simulink model "LQR_Hardware"  (R2022b)
settings: Solver=ode1  StartTime=0.0  StopTime=inf  FixedStep=0.001  RelTol=1e-3
values from neighbouring files (symbols this model uses):
  KK = lqr(A,B,Q,R)    [Init_Setup_LQRArd.m]    (also in Parameters.m)
libraries: arduinolib x4, arduinosensorlib x2
settings Model: ExtModeTrigDuration=2  Creator=sokse  LastModifiedBy=sokse
settings OptimizationCC: EnhancedBackFolding=on  PassReuseOutputArgsAs=Individual arguments  ZeroExternalMemoryAtStartup=off  ZeroInternalMemoryAtStartup=off  MaxStackSize=64  OptimizeBlockOrder=speed  DifferentSizesBufferReuse=on  OptimizationCustomize=off  EfficientTunableParamExpr=on
settings DebuggingCC: ParameterTunabilityLossMsg=error
settings HardwareCC: ProdBitPerInt=16  ProdBitPerPointer=16  ProdBitPerSizeT=16  ProdBitPerPtrDiffT=16  ProdLargestAtomicFloat=None  ProdWordSize=8  ProdHWDeviceType=Atmel->AVR
settings SFSimCC: MATLABDynamicMemAlloc=off
settings RTWCC: Description=Embedded Coder  SystemTargetFile=ert.tlc  HardwareBoard=Arduino Mega 2560  TLCOptions=-aInlineSetEventsForThisBaseRateFcn=TLC_FALSE -aSuppressMultiTaskScheduler=TLC_FALSE -aRateBasedStepFcn=1  TemplateMakefile=ert_default_tmf  Toolchain=Arduino AVR  BuildConfiguration=Faster Runs
settings CodeAppCC: ForceParamTrailComments=on  IgnoreCustomStorageClasses=off  OperatorAnnotations=on  SimulinkDataObjDesc=on  SFDataObjDesc=on  InsertBlockDesc=on
settings ERTTargetCC: SupportContinuousTime=on  SupportVariableSizeSignals=on  ExtModeTransport=3  ExtModeStaticAlloc=on  ExtModeAutomaticAllocSize=off  ExtModeStaticAllocSize=2048  ExtModeMexFile=ext_xcp  ExtModeIntrfLevel=Level2 - Open

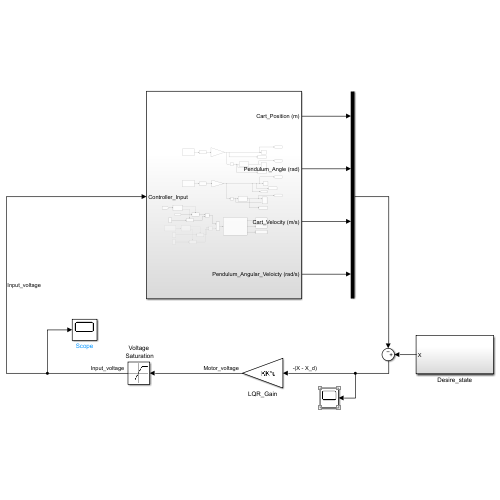
[thumbnail: Simulink's stored preview of the top-level diagram]
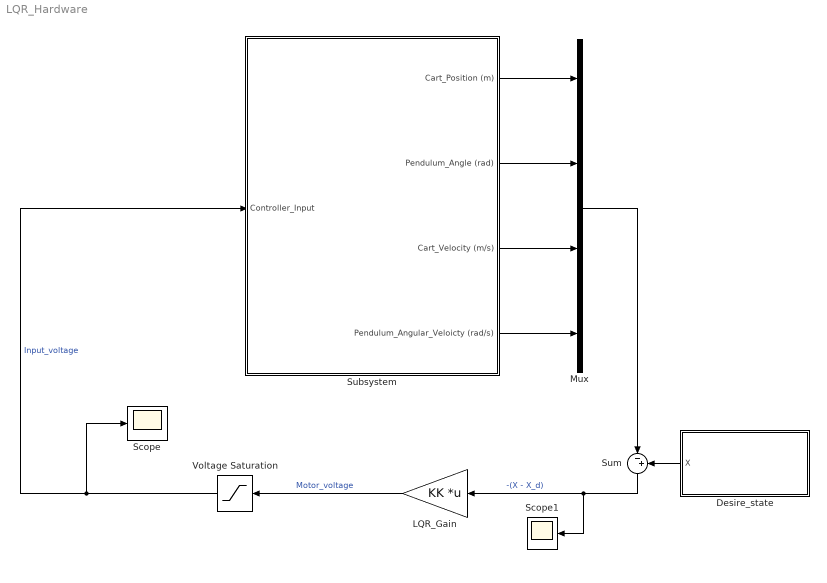
== system LQR_Hardware ==
  Desire_state : Subsystem
  LQR_Gain : Gain  Gain=KK  Multiplication=Matrix(K*u)
  Mux : Mux
  Scope : Scope
  Scope1 : Scope
  Subsystem : Subsystem
  Sum : Sum  Inputs=|-+
  Voltage Saturation : Saturate  UpperLimit=12  LowerLimit=-12
  wires:
  Voltage Saturation/1 -> Scope/1, Subsystem/1(Controller_Input)  "Input_voltage"
  Sum/1 -> Scope1/1, LQR_Gain/1  "-(X - X_d)"
  Desire_state/1(X) -> Sum/2
  LQR_Gain/1 -> Voltage Saturation/1  "Motor_voltage"
  Subsystem/1(Cart_Position (m)) -> Mux/1
  Subsystem/2(Pendulum_Angle (rad)) -> Mux/2
  Subsystem/3(Cart_Velocity (m/s)) -> Mux/3
  Subsystem/4(Pendulum_Angular_Veloicty (rad/s)) -> Mux/4
  Mux/1 -> Sum/1

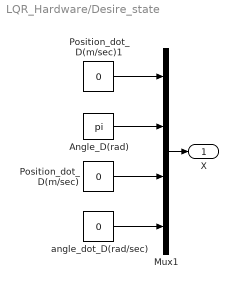
== system LQR_Hardware/Desire_state ==
  Angle_D(rad) : Constant  Value=pi
  Mux1 : Mux
  Position_dot_D(m/sec) : Constant  Value=0
  Position_dot_D(m/sec)1 : Constant  Value=0
  angle_dot_D(rad/sec) : Constant  Value=0
  X : Outport  VectorParamsAs1DForOutWhenUnconnected=off
  wires:
  Position_dot_D(m/sec)1/1 -> Mux1/1
  Angle_D(rad)/1 -> Mux1/2
  angle_dot_D(rad/sec)/1 -> Mux1/4
  Position_dot_D(m/sec)/1 -> Mux1/3
  Mux1/1 -> X/1

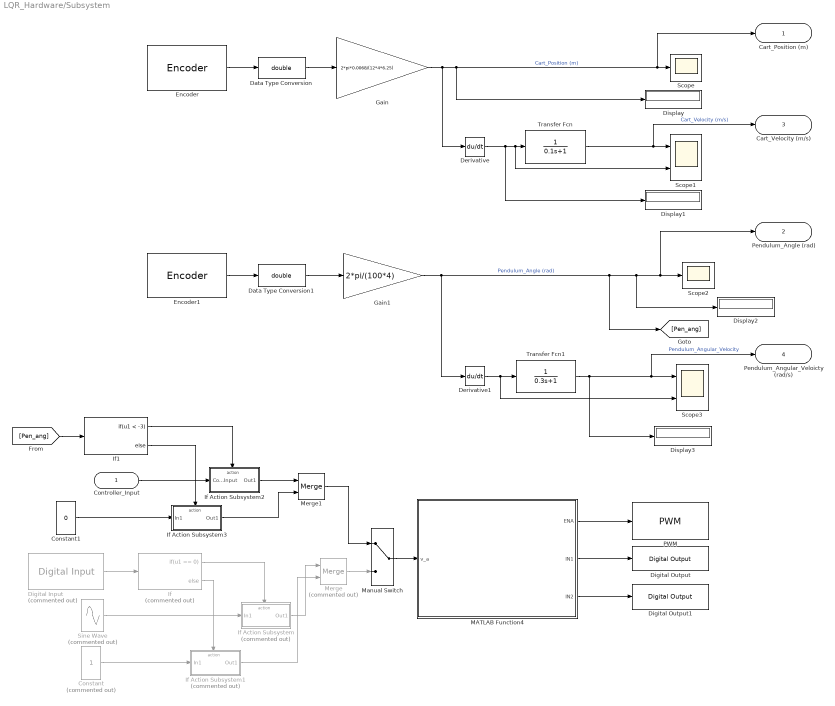
== system LQR_Hardware/Subsystem ==
  Controller_Input : Inport
  Constant : Constant  Commented=on
  Constant1 : Constant  Value=0
  Data Type Conversion : DataTypeConversion  OutDataTypeStr=double  SaturateOnIntegerOverflow=off  RndMeth=Floor
  Data Type Conversion1 : DataTypeConversion  OutDataTypeStr=double  SaturateOnIntegerOverflow=off  RndMeth=Floor
  Derivative : Derivative
  Derivative1 : Derivative
  Digital Input : arduinolib/Digital Input  Commented=on  pinNumber=13  mode=Input Pullup  Direction=input  SampleTime=0.001  blockPlatform=arduino
  Digital Output : arduinolib/Digital Output  pinNumber=9  Direction=output  blockPlatform=arduino
  Digital Output1 : arduinolib/Digital Output  pinNumber=10  Direction=output  blockPlatform=arduino
  Display{,1..3} (4 alike) : Display
  Encoder : arduinosensorlib/Encoder  InputA=2  InputB=3  Mode=No reset  SampleTime=0.01
  Encoder1 : arduinosensorlib/Encoder  InputA=20  InputB=21  Mode=No reset  SampleTime=0.01
  Gain : Gain  Gain=2*pi*0.0068/(12*4*6.25)
  Gain1 : Gain  Gain=2*pi/(100*4)
  If : If  Commented=on  IfExpression=u1 == 0
  If Action Subsystem : Subsystem  Commented=on  TreatAsAtomicUnit=on
  If Action Subsystem1 : Subsystem  Commented=on  TreatAsAtomicUnit=on
  If Action Subsystem2 : Subsystem  TreatAsAtomicUnit=on
  If Action Subsystem3 : Subsystem  TreatAsAtomicUnit=on
  If1 : If  IfExpression=u1 < -3
  MATLAB Function4 : MATLAB Function  TreatAsAtomicUnit=on
  Manual Switch : ManualSwitch
  Merge : Merge  Commented=on
  Merge1 : Merge
  PWM : arduinolib/PWM  pinNumber=11  frequencyType=Default  desiredFrequency=490.2  achievableFrequency=490.2
  Scope : Scope
  Scope1 : Scope  NumInputPorts=2
  Scope2 : Scope
  Scope3 : Scope  NumInputPorts=2
  Sine Wave : Sin  Commented=on  Amplitude=8  Frequency=4  SampleTime=0
  Transfer Fcn : TransferFcn  Denominator=[0.1 1]
  Transfer Fcn1 : TransferFcn  Denominator=[0.3 1]
  Cart_Position (m) : Outport
  Pendulum_Angle (rad) : Outport  Port=2
  Cart_Velocity (m/s) : Outport  Port=3
  Pendulum_Angular_Veloicty (rad/s) : Outport  Port=4
  wires:
  Encoder1/1 -> Data Type Conversion1/1
  MATLAB Function4/3(IN2) -> Digital Output1/1
  Gain/1 -> Derivative/1, Display/1, Cart_Position (m)/1, Scope/1  "Cart_Position (m)"
  Transfer Fcn1/1 -> Display3/1, Pendulum_Angular_Veloicty (rad/s)/1, Scope3/1  "Pendulum_Angular_Velocity"
  Derivative/1 -> Display1/1, Scope1/2, Transfer Fcn/1
  Derivative1/1 -> Scope3/2, Transfer Fcn1/1
  Encoder/1 -> Data Type Conversion/1
  Transfer Fcn/1 -> Cart_Velocity (m/s)/1, Scope1/1  "Cart_Velocity (m/s)"
  Data Type Conversion/1 -> Gain/1
  MATLAB Function4/2(IN1) -> Digital Output/1
  MATLAB Function4/1(ENA) -> PWM/1
  Manual Switch/1 -> MATLAB Function4/1(v_a)
  Merge/1 -> Manual Switch/2
  If/1 -> If Action Subsystem/Action
  Digital Input/1 -> If/1
  Sine Wave/1 -> If Action Subsystem/1(In1)
  If/2 -> If Action Subsystem1/Action
  Constant/1 -> If Action Subsystem1/1(In1)
  If Action Subsystem/1(Out1) -> Merge/1
  If Action Subsystem1/1(Out1) -> Merge/2
  Gain1/1 -> [Pen_ang], Display2/1, Pendulum_Angle (rad)/1, Scope2/1, Derivative1/1  "Pendulum_Angle (rad)"
  [Pen_ang] -> If1/1
  Data Type Conversion1/1 -> Gain1/1
  If1/1 -> If Action Subsystem2/Action
  Controller_Input/1 -> If Action Subsystem2/1(Controller_Input)
  If Action Subsystem2/1(Out1) -> Merge1/1
  Constant1/1 -> If Action Subsystem3/1(In1)
  If1/2 -> If Action Subsystem3/Action
  If Action Subsystem3/1(Out1) -> Merge1/2
  Merge1/1 -> Manual Switch/1

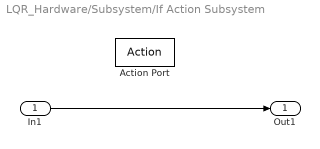
== system LQR_Hardware/Subsystem/If Action Subsystem ==
  In1 : Inport
  Action Port : ActionPort  ActionPortLabel=if(u1 == 0)
  Out1 : Outport
  wires:
  In1/1 -> Out1/1

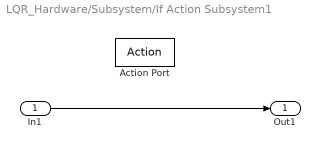
== system LQR_Hardware/Subsystem/If Action Subsystem1 ==
  In1 : Inport
  Action Port : ActionPort  ActionPortLabel=else
  Out1 : Outport
  wires:
  In1/1 -> Out1/1

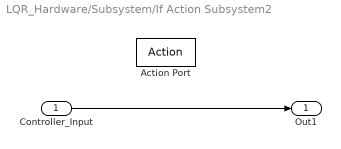
== system LQR_Hardware/Subsystem/If Action Subsystem2 ==
  Controller_Input : Inport
  Action Port : ActionPort  ActionPortLabel=if(u1 < -3)
  Out1 : Outport
  wires:
  Controller_Input/1 -> Out1/1

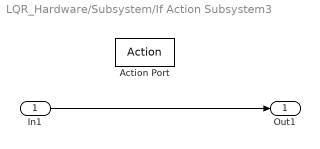
== system LQR_Hardware/Subsystem/If Action Subsystem3 ==
  In1 : Inport
  Action Port : ActionPort  ActionPortLabel=else
  Out1 : Outport
  wires:
  In1/1 -> Out1/1

== matlab function LQR_Hardware/Subsystem/MATLAB Function4 ==
  data: v_a input; ENA output; IN1 output; IN2 output
function [ENA,IN1,IN2] = fcn(v_a)

vmax = 12;
pwm_cal = v_a*254/vmax;

if pwm_cal > 0
   
    ENA = pwm_cal;
    IN1 = 0;
    IN2 = 1;
elseif pwm_cal < 0
   
    ENA = abs(pwm_cal);
    IN1 = 1;
    IN2 = 0;
else
    ENA = 0;
    IN1 = 0;
    IN2 = 0;
   
end
